simulink model "z335c_Sim"  (Simulink 7.1)
settings: Solver=ode45  StartTime=0.0  StopTime=15.0  RelTol=1e-3
undefined symbols (not defined in the file or in its folder): Stanje_1
settings Model: Creator=mestar  LastModifiedBy=mestar

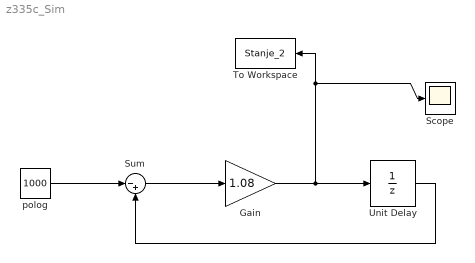
== system z335c_Sim ==
  Gain : Gain  Gain=1.08  ParameterDataType=sfix(16)  ParameterScaling=2^0  OutDataType=sfix(16)  OutScaling=2^0
  Scope : Scope
      settings: TimeRange=15
  Sum : Sum  Inputs=|-+  OutDataType=sfix(16)  OutScaling=2^0
  To Workspace : ToWorkspace  VariableName=Stanje_2  SampleTime=-1  SaveFormat=Array
  Unit Delay : UnitDelay  X0=Stanje_1(15)
  polog : Constant  Value=1000  OutDataType=sfix(16)  OutScaling=2^0
  wires:
  polog/1 -> Sum/1
  Sum/1 -> Gain/1
  Gain/1 -> Unit Delay/1, To Workspace/1, Scope/1
  Unit Delay/1 -> Sum/2
